simulink model "TireTestRig"  (R2020b)
settings: Solver=ode1  StartTime=0.0  StopTime=Tf  FixedStep=Ts  RelTol=1e-3  EnableMultiTasking=on
values from neighbouring files (symbols this model uses):
  Fz_forced = 1    [Main.m]
  p1 = 20    [Main.m]
  p2 = tire_data.UNLOADED_RADIUS    [Main.m]
  p3 = 9    [Main.m]
  p4 = 0.11    [Main.m]
  p5 = 6    [Main.m]
  p6 = tire_data.WIDTH/2    [Main.m]
  p7 = 1    [Main.m]
  p8 = 0    [Main.m]
  road_file = '../files_rdf/sample.rdf'    [Main.m]
  test_name = 'sine_thetaX'    [Main.m]
  tire_data = TIR_read('205_60_R15__left_debug.tir')    [Main.m]
  Ts = 1e-3    (= 0.001)    [Main.m]
undefined symbols (not defined in the file or in its folder): DiscIntNeverNeededParam, en_pressure, en_theta_x, en_theta_y, en_theta_z, en_x, en_y, en_z, inputs
libraries: RF_transformations x9, simulink x7, pid_lib x1, tire x1
settings Model: PacingRate=0.028000  Creator=matteolarcher  LastModifiedBy=matteolarcher
settings SolverCC: ConcurrentTasks=on
settings DataIOCC: SaveFormat=Array  ReturnWorkspaceOutputs=off

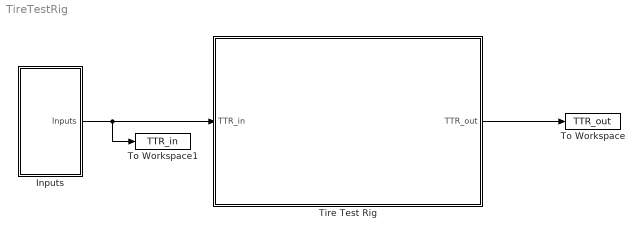
== system TireTestRig ==
  Inputs : Subsystem
  Tire Test Rig : Subsystem
  To Workspace : ToWorkspace  VariableName=TTR_out  SaveFormat=Timeseries  SampleTime=-1
  To Workspace1 : ToWorkspace  VariableName=TTR_in  SaveFormat=Timeseries  SampleTime=-1
  wires:
  Inputs/1(Inputs) -> To Workspace1/1, Tire Test Rig/1(TTR_in)
  Tire Test Rig/1(TTR_out) -> To Workspace/1

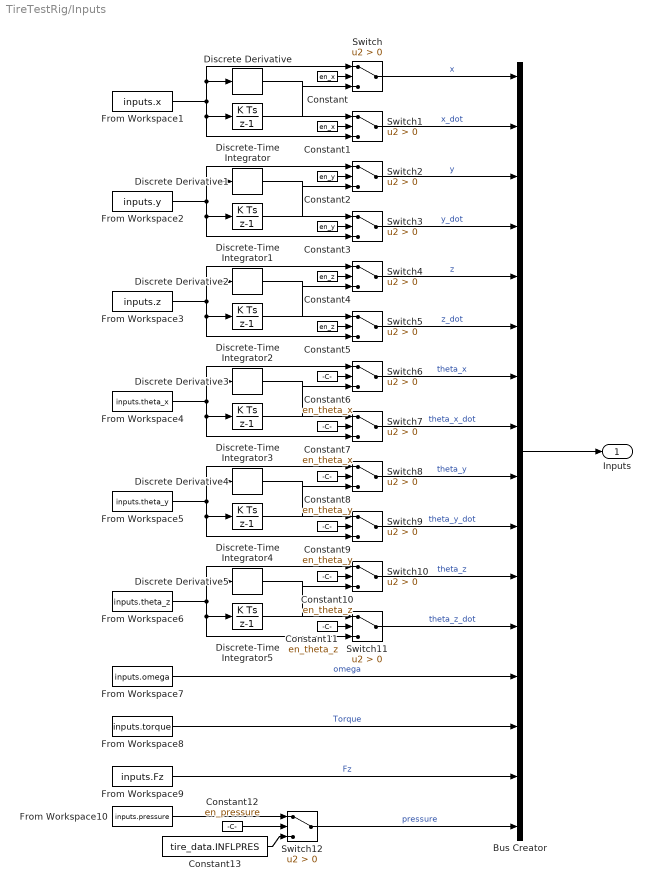
== system TireTestRig/Inputs ==
  Bus Creator : BusCreator  Inputs=16
  Constant : Constant  Value=en_x
  Constant1 : Constant  Value=en_x
  Constant10 : Constant  Value=en_theta_z
  Constant11 : Constant  Value=en_theta_z
  Constant12 : Constant  Value=en_pressure
  Constant13 : Constant  Value=tire_data.INFLPRES
  Constant2 : Constant  Value=en_y
  Constant3 : Constant  Value=en_y
  Constant4 : Constant  Value=en_z
  Constant5 : Constant  Value=en_z
  Constant6 : Constant  Value=en_theta_x
  Constant7 : Constant  Value=en_theta_x
  Constant8 : Constant  Value=en_theta_y
  Constant9 : Constant  Value=en_theta_y
  Discrete Derivative{,1..5} (6 alike) : simulink/Discrete/Discrete Derivative  gainval=1.0  ICPrevScaledInput=0.0  OutMin=[]  OutMax=[]  OutDataType=fixdt(1, 16)  OutScaling=2^-10  DoSatur=off
  Discrete-Time Integrator : DiscreteIntegrator  InitialCondition=inputs.x0  SampleTime=-1  ICPrevOutput=DiscIntNeverNeededParam  ICPrevScaledInput=DiscIntNeverNeededParam
  Discrete-Time Integrator1 : DiscreteIntegrator  InitialCondition=inputs.y0  SampleTime=-1  ICPrevOutput=DiscIntNeverNeededParam  ICPrevScaledInput=DiscIntNeverNeededParam
  Discrete-Time Integrator2 : DiscreteIntegrator  InitialCondition=inputs.z0  SampleTime=-1  ICPrevOutput=DiscIntNeverNeededParam  ICPrevScaledInput=DiscIntNeverNeededParam
  Discrete-Time Integrator3 : DiscreteIntegrator  InitialCondition=inputs.theta_x0  SampleTime=-1  ICPrevOutput=DiscIntNeverNeededParam  ICPrevScaledInput=DiscIntNeverNeededParam
  Discrete-Time Integrator4 : DiscreteIntegrator  InitialCondition=inputs.theta_y0  SampleTime=-1  ICPrevOutput=DiscIntNeverNeededParam  ICPrevScaledInput=DiscIntNeverNeededParam
  Discrete-Time Integrator5 : DiscreteIntegrator  InitialCondition=inputs.theta_z0  SampleTime=-1  ICPrevOutput=DiscIntNeverNeededParam  ICPrevScaledInput=DiscIntNeverNeededParam
  From Workspace1 : FromWorkspace  VariableName=inputs.x
  From Workspace10 : FromWorkspace  VariableName=inputs.pressure
  From Workspace2 : FromWorkspace  VariableName=inputs.y
  From Workspace3 : FromWorkspace  VariableName=inputs.z
  From Workspace4 : FromWorkspace  VariableName=inputs.theta_x
  From Workspace5 : FromWorkspace  VariableName=inputs.theta_y
  From Workspace6 : FromWorkspace  VariableName=inputs.theta_z
  From Workspace7 : FromWorkspace  VariableName=inputs.omega
  From Workspace8 : FromWorkspace  VariableName=inputs.torque
  From Workspace9 : FromWorkspace  VariableName=inputs.Fz
  Switch{,1..12} (13 alike) : Switch  Criteria=u2 > Threshold
  Inputs : Outport
  wires:
  Bus Creator/1 -> Inputs/1
  Switch/1 -> Bus Creator/1  "x"
  Discrete Derivative/1 -> Switch1/1
  Switch1/1 -> Bus Creator/2  "x_dot"
  From Workspace1/1 -> Switch/1, Discrete Derivative/1, Switch1/3, Discrete-Time Integrator/1
  Discrete-Time Integrator/1 -> Switch/3
  Constant/1 -> Switch/2
  Constant1/1 -> Switch1/2
  Constant3/1 -> Switch3/2
  Constant2/1 -> Switch2/2
  Discrete-Time Integrator1/1 -> Switch2/3
  From Workspace2/1 -> Discrete-Time Integrator1/1, Switch3/3, Discrete Derivative1/1, Switch2/1
  Switch3/1 -> Bus Creator/4  "y_dot"
  Discrete Derivative1/1 -> Switch3/1
  Switch2/1 -> Bus Creator/3  "y"
  Switch4/1 -> Bus Creator/5  "z"
  Discrete Derivative2/1 -> Switch5/1
  Switch5/1 -> Bus Creator/6  "z_dot"
  From Workspace3/1 -> Switch4/1, Discrete Derivative2/1, Switch5/3, Discrete-Time Integrator2/1
  Discrete-Time Integrator2/1 -> Switch4/3
  Constant4/1 -> Switch4/2
  Constant5/1 -> Switch5/2
  Constant11/1 -> Switch11/2
  Constant10/1 -> Switch10/2
  Discrete-Time Integrator5/1 -> Switch10/3
  From Workspace6/1 -> Discrete-Time Integrator5/1, Switch11/3, Discrete Derivative5/1, Switch10/1
  Switch11/1 -> Bus Creator/12  "theta_z_dot"
  Discrete Derivative5/1 -> Switch11/1
  Switch10/1 -> Bus Creator/11  "theta_z"
  Switch8/1 -> Bus Creator/9  "theta_y"
  Discrete Derivative4/1 -> Switch9/1
  Switch9/1 -> Bus Creator/10  "theta_y_dot"
  From Workspace5/1 -> Switch8/1, Discrete Derivative4/1, Switch9/3, Discrete-Time Integrator4/1
  Discrete-Time Integrator4/1 -> Switch8/3
  Constant8/1 -> Switch8/2
  Constant9/1 -> Switch9/2
  Constant7/1 -> Switch7/2
  Constant6/1 -> Switch6/2
  Discrete-Time Integrator3/1 -> Switch6/3
  From Workspace4/1 -> Discrete-Time Integrator3/1, Switch7/3, Discrete Derivative3/1, Switch6/1
  Switch7/1 -> Bus Creator/8  "theta_x_dot"
  Discrete Derivative3/1 -> Switch7/1
  Switch6/1 -> Bus Creator/7  "theta_x"
  From Workspace7/1 -> Bus Creator/13  "omega"
  From Workspace8/1 -> Bus Creator/14  "Torque"
  From Workspace9/1 -> Bus Creator/15  "Fz"
  From Workspace10/1 -> Switch12/1
  Constant12/1 -> Switch12/2
  Constant13/1 -> Switch12/3
  Switch12/1 -> Bus Creator/16  "pressure"

== system TireTestRig/Tire Test Rig ==
  note: in sin ThetaY anomalia pc e normale
      |
      | libreria macroblocchi
      |
      | controllo per 0 long slip
  TTR_in : Inport
  TTR_outputs : BusCreator  Inputs=3
  TireTestRig : Subsystem  TreatAsAtomicUnit=on
  TTR_out : Outport
  wires:
  TTR_outputs/1 -> TTR_out/1
  TTR_in/1 -> TireTestRig/1(inputs)
  TireTestRig/1(Tire Bus) -> TTR_outputs/1  "Tire Bus"
  TireTestRig/2(ENVE Bus) -> TTR_outputs/2  "ENVE Bus"
  TireTestRig/3(Actuator Bus) -> TTR_outputs/3  "Actuator Bus"

== system TireTestRig/Tire Test Rig/TireTestRig ==
  inputs : Inport
  ENVE : Subsystem
  Graphics : Subsystem
  Rig Actuator : Subsystem
  Tire : Subsystem
  Tire Bus : Outport
  ENVE Bus : Outport  Port=2
  Actuator Bus : Outport  Port=3
  wires:
  inputs/1 -> Tire/3(Inputs), Rig Actuator/2(inputs)
  Tire/1(Tire Bus) -> Graphics/1(Tire Bus), Tire Bus/1, Rig Actuator/1(tire Bus)
  Rig Actuator/1(Actuator Bus) -> Actuator Bus/1, Graphics/3(Actuator Bus), Tire/2(Actuator Bus), ENVE/1(Actuator Bus)
  ENVE/1(ENVE Bus) -> ENVE Bus/1, Graphics/2(ENVE Bus), Tire/1(ENVE Bus)

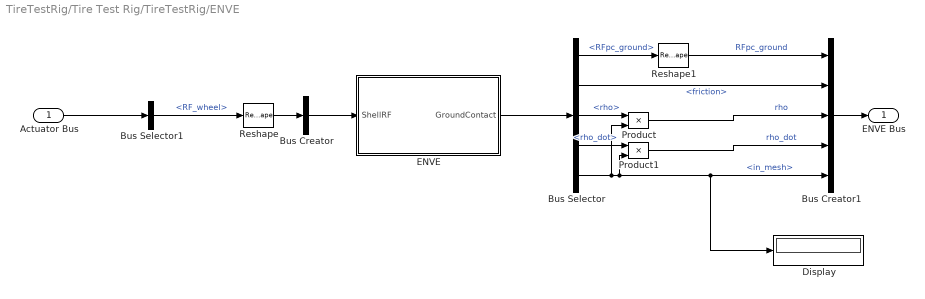
== system TireTestRig/Tire Test Rig/TireTestRig/ENVE ==
  Actuator Bus : Inport
  Bus Creator : BusCreator  Inputs=1  OutDataTypeStr=Bus: shellRF
      settings: InheritFromInputs=off
  Bus Creator1 : BusCreator  Inputs=5
  Bus Selector : BusSelector  OutputSignals=RFpc_ground,friction,rho,rho_dot,in_mesh
  Bus Selector1 : BusSelector  OutputSignals=RF_wheel
  Display : Display
  ENVE : Subsystem  mask{SParameter1=p1, SParameter2=p2, SParameter3=p3, SParameter4=p4, SParameter5=p5, SParameter6=p6, SParameter7=p7, SParameter8=p8}
      mask prompts: SParameter1 "Ribs number"; SParameter2 "Shell radius on x axis (m)"; SParameter3 "Shell curve degree for x axis"; SParameter4 "Shell radius on y axis (m)"; SParameter5 "Shell curve degree for y axis"; SParameter6 "Shell half width on y axis (m)"; SParameter7 "enveloping method"; SParameter8 "flat_enable"
      mask TypeOptions SParameter1: sfun_ENVE_VIRTUALTESTBENCH/SParameter1
      mask TypeOptions SParameter2: sfun_ENVE_VIRTUALTESTBENCH/SParameter2
      mask TypeOptions SParameter3: sfun_ENVE_VIRTUALTESTBENCH/SParameter3
      mask TypeOptions SParameter4: sfun_ENVE_VIRTUALTESTBENCH/SParameter4
      mask TypeOptions SParameter5: sfun_ENVE_VIRTUALTESTBENCH/SParameter5
      mask TypeOptions SParameter6: sfun_ENVE_VIRTUALTESTBENCH/SParameter6
      mask TypeOptions SParameter7: sfun_ENVE_VIRTUALTESTBENCH/SParameter7
      mask TypeOptions SParameter8: sfun_ENVE_VIRTUALTESTBENCH/SParameter8
  Product : Product
  Product1 : Product
  Reshape : Reshape
  Reshape1 : Reshape  OutputDimensionality=Customize  OutputDimensions=[4,4]
  ENVE Bus : Outport
  wires:
  Product1/1 -> Bus Creator1/4  "rho_dot"
  Bus Selector/5 -> Product/2, Display/1, Bus Creator1/5, Product1/2  "<in_mesh>"
  Reshape1/1 -> Bus Creator1/1  "RFpc_ground"
  Bus Creator/1 -> ENVE/1(ShellRF)
  Product/1 -> Bus Creator1/3  "rho"
  ENVE/1(GroundContact) -> Bus Selector/1
  Bus Selector/2 -> Bus Creator1/2  "<friction>"
  Bus Selector/1 -> Reshape1/1  "<RFpc_ground>"
  Actuator Bus/1 -> Bus Selector1/1
  Reshape/1 -> Bus Creator/1
  Bus Selector/3 -> Product/1  "<rho>"
  Bus Selector/4 -> Product1/1  "<rho_dot>"
  Bus Selector1/1 -> Reshape/1  "<RF_wheel>"
  Bus Creator1/1 -> ENVE Bus/1

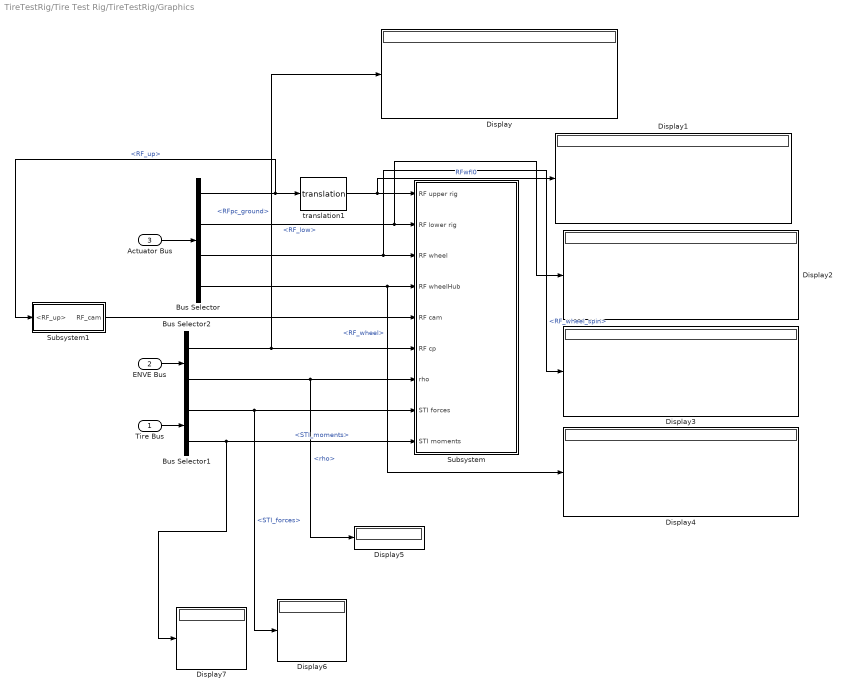
== system TireTestRig/Tire Test Rig/TireTestRig/Graphics ==
  Tire Bus : Inport
  ENVE Bus : Inport  Port=2
  Actuator Bus : Inport  Port=3
  Bus Selector : BusSelector  OutputSignals=RF_up,RF_low,RF_wheel_spin,RF_wheel
  Bus Selector1 : BusSelector  OutputSignals=STI_forces,STI_moments
  Bus Selector2 : BusSelector  OutputSignals=RFpc_ground,rho
  Display{,1..7} (8 alike) : Display
  Subsystem : Subsystem  mask{sample_time=Ts*100, tire_data=tire_data, road_file=road_file, rig_up_stl='rig_up.stl', rig_up_stl_scale=1e-3, rig_low_stl='rig_low.stl', rig_low_stl_scale=1e-3, wheel_stl={'SHELL',p1,p2,p3,p4,p5,p6}, wheel_stl_scale=1, en_trace_wheel=off, en_trace_cp=off, en_RF_wheel=on, en_RF_cp=on, en_RF_wheelHub=on, en_normal=on, en_forces=on, en_moments=on, save_gif=on, gif_folder=['./outputs/', test_name, '/GIF']}
      mask prompts: sample_time "sample time"; road_file "road file"; rig_up_stl "rig upper stl"; rig_up_stl_scale "rig upper stl scaling factor"; rig_low_stl "rig lower stl"; rig_low_stl_scale "rig lower stl scaling factor"; wheel_stl "wheel stl"; wheel_stl_scale "wheel stl scaling factor"; en_trace_wheel "enable wheel trace"; en_trace_cp "enable contact point trace"; en_RF_wheel "enable RF wheel"; en_RF_cp "enable RF contact point"; en_RF_wheelHub "enable RF wheel hub"; en_normal "enable normal vector"; en_forces "enable STI forces"; en_moments "enable STI moments"; save_gif "Save GIF"; gif_folder "GIF folder"
      mask init:
      | % create stl from shell geometry
      | if iscell(wheel_stl) && strcmp(wheel_stl{1}, 'SHELL')
      |     S = enve_shell(wheel_stl{2},wheel_stl{3},wheel_stl{4},wheel_stl{5},wheel_stl{6},wheel_stl{7});
      |     mesh = S.meshShell;
      |     surf2stl('./tmp/SHELL.stl',mesh.X,mesh.Y,mesh.Z,'ascii');
      |     wheel_stl = 'SHELL.stl';
      |     en_realdim_scaling = 0;
      | else
      |     en_realdim_scaling = 1;
      | end
      mask TypeOptions sample_time:
      | Level-2 MATLAB
      | S-Function1/sample_time
      mask TypeOptions tire_data:
      | Level-2 MATLAB
      | S-Function1/tire_data
      mask TypeOptions road_file:
      | Level-2 MATLAB
      | S-Function1/road_file
      mask TypeOptions rig_up_stl:
      | Level-2 MATLAB
      | S-Function1/rig_up_stl
      mask TypeOptions rig_up_stl_scale:
      | Level-2 MATLAB
      | S-Function1/rig_up_stl_scale
      mask TypeOptions rig_low_stl:
      | Level-2 MATLAB
      | S-Function1/rig_low_stl
      mask TypeOptions rig_low_stl_scale:
      | Level-2 MATLAB
      | S-Function1/rig_low_stl_scale
      mask TypeOptions wheel_stl:
      | Level-2 MATLAB
      | S-Function1/wheel_stl
      mask TypeOptions wheel_stl_scale:
      | Level-2 MATLAB
      | S-Function1/wheel_stl_scale
      mask TypeOptions en_trace_wheel:
      | Level-2 MATLAB
      | S-Function1/en_trace_wheel
      mask TypeOptions en_trace_cp:
      | Level-2 MATLAB
      | S-Function1/en_trace_cp
      mask TypeOptions en_RF_wheel:
      | Level-2 MATLAB
      | S-Function1/en_RF_wheel
      mask TypeOptions en_RF_cp:
      | Level-2 MATLAB
      | S-Function1/en_RF_cp
      mask TypeOptions en_RF_wheelHub:
      | Level-2 MATLAB
      | S-Function1/en_RF_wheelHub
      mask TypeOptions en_normal:
      | Level-2 MATLAB
      | S-Function1/en_normal
      mask TypeOptions en_forces:
      | Level-2 MATLAB
      | S-Function1/en_forces
      mask TypeOptions en_moments:
      | Level-2 MATLAB
      | S-Function1/en_moments
      mask TypeOptions save_gif:
      | Level-2 MATLAB
      | S-Function1/save_gif
      mask TypeOptions gif_folder:
      | Level-2 MATLAB
      | S-Function1/gif_folder
      mask DialogControl Container3 Prompt: GIF
  Subsystem1 : Subsystem  mask{xt=1, yt=-0, zt=0.2}
  translation1 : RF_transformations/translation  xt=0  yt=0.3+0.075  zt=0.3
  wires:
  Bus Selector/2 -> Display2/1, Subsystem/2(RF lower rig)  "<RF_low>"
  translation1/1 -> Display1/1, Subsystem/1(RF upper rig)  "RFwfl0"
  Bus Selector/3 -> Display3/1, Subsystem/3(RF wheel)  "<RF_wheel_spin>"
  Actuator Bus/1 -> Bus Selector/1
  Bus Selector/1 -> Subsystem1/1(<RF_up>), translation1/1  "<RF_up>"
  Tire Bus/1 -> Bus Selector1/1
  ENVE Bus/1 -> Bus Selector2/1
  Bus Selector2/1 -> Display/1, Subsystem/6(RF cp)  "<RFpc_ground>"
  Bus Selector2/2 -> Display5/1, Subsystem/7(rho)  "<rho>"
  Bus Selector1/1 -> Display6/1, Subsystem/8(STI forces)  "<STI_forces>"
  Bus Selector1/2 -> Display7/1, Subsystem/9(STI moments)  "<STI_moments>"
  Bus Selector/4 -> Display4/1, Subsystem/4(RF wheelHub)  "<RF_wheel>"
  Subsystem1/1(RF_cam) -> Subsystem/5(RF cam)

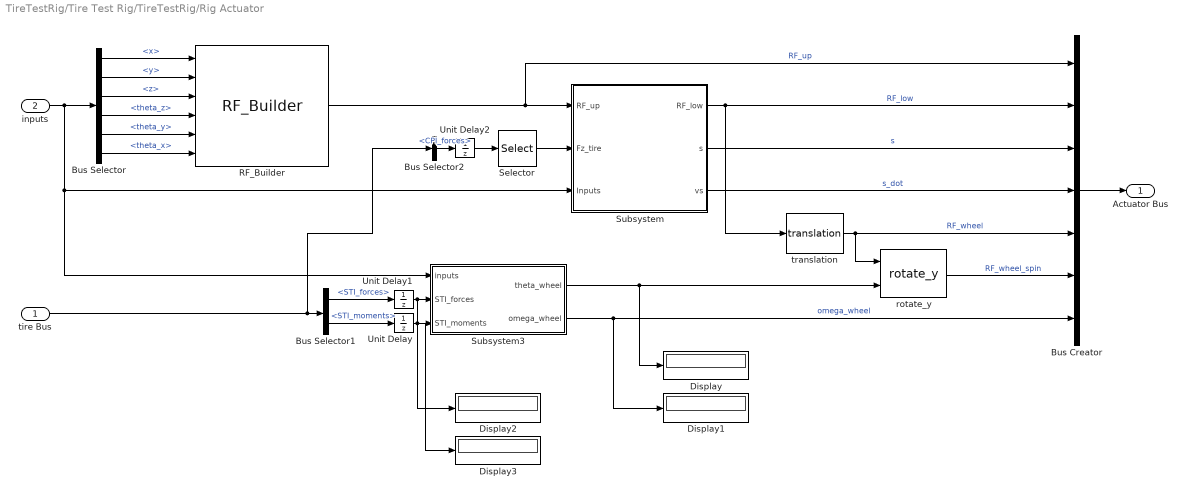
== system TireTestRig/Tire Test Rig/TireTestRig/Rig Actuator ==
  tire Bus : Inport
  inputs : Inport  Port=2
  Bus Creator : BusCreator  Inputs=7
  Bus Selector : BusSelector  OutputSignals=x,y,z,theta_z,theta_y,theta_x
  Bus Selector1 : BusSelector  OutputSignals=STI_forces,STI_moments
  Bus Selector2 : BusSelector  OutputSignals=CPI_forces
  Display{,1..3} (4 alike) : Display
  RF_Builder : RF_transformations/RF_Builder  order_selector=['Z','Y','X']
  Selector : Selector  InputPortWidth=3  IndexOptions=Index vector (dialog)  Indices=[3]  OutputSizes=1
  Subsystem : Subsystem  Variant=on  VariantControl=Choice
  Subsystem3 : Subsystem
  Unit Delay : UnitDelay  SampleTime=-1  HasFrameUpgradeWarning=on
  Unit Delay1 : UnitDelay  SampleTime=-1  HasFrameUpgradeWarning=on
  Unit Delay2 : UnitDelay  SampleTime=-1  HasFrameUpgradeWarning=on
  rotate_y : RF_transformations/rotate_y  SystemSampleTime=-1  VariantActivationTime=update diagram  Latency=0  AutoFrameSizeCalculation=off
  translation : RF_transformations/translation  xt=0  yt=0  zt=0
  Actuator Bus : Outport
  wires:
  Subsystem/2(s) -> Bus Creator/3  "s"
  Subsystem/3(vs) -> Bus Creator/4  "s_dot"
  Selector/1 -> Subsystem/2(Fz_tire)
  Subsystem/1(RF_low) -> translation/1, Bus Creator/2  "RF_low"
  Bus Selector2/1 -> Unit Delay2/1  "<CPI_forces>"
  RF_Builder/1 -> Subsystem/1(RF_up), Bus Creator/1  "RF_up"
  Bus Selector/5 -> RF_Builder/5  "<theta_y>"
  Bus Selector/4 -> RF_Builder/4  "<theta_z>"
  Bus Selector/6 -> RF_Builder/6  "<theta_x>"
  Bus Selector/3 -> RF_Builder/3  "<z>"
  Bus Selector/2 -> RF_Builder/2  "<y>"
  Bus Selector/1 -> RF_Builder/1  "<x>"
  inputs/1 -> Bus Selector/1, Subsystem3/1(inputs), Subsystem/3(Inputs)
  rotate_y/1 -> Bus Creator/6  "RF_wheel_spin"
  translation/1 -> rotate_y/1, Bus Creator/5  "RF_wheel"
  Subsystem3/1(theta_wheel) -> Display/1, rotate_y/2
  Subsystem3/2(omega_wheel) -> Display1/1, Bus Creator/7  "omega_wheel"
  Bus Selector1/2 -> Unit Delay/1  "<STI_moments>"
  Bus Selector1/1 -> Unit Delay1/1  "<STI_forces>"
  tire Bus/1 -> Bus Selector2/1, Bus Selector1/1
  Bus Creator/1 -> Actuator Bus/1
  Unit Delay/1 -> Display3/1, Subsystem3/3(STI_moments)
  Unit Delay1/1 -> Display2/1, Subsystem3/2(STI_forces)
  Unit Delay2/1 -> Selector/1

== system TireTestRig/Tire Test Rig/TireTestRig/Tire ==
  ENVE Bus : Inport
  Actuator Bus : Inport  Port=2
  Inputs : Inport  Port=3
  Bus Creator : BusCreator  Inputs=7
  Display : Display
  Display1 : Display
  Display2 : Display
  My_Tire_programmable : tire/My_Tire_programmable  Ts_tire=-1  tmp_tire_data=tire_data  enabled_rewind_tire=off  PauseResume=0  USE_MODE=tire_use_mode  pressure_from=tire pressure from input port  tire_p=1  Fz_flag=Fz_forced
  Subsystem1 : Subsystem
  Tire Bus : Outport
  wires:
  My_Tire_programmable/1 -> Bus Creator/1  "CPI_forces"
  My_Tire_programmable/2 -> Bus Creator/2  "CPI_moments"
  My_Tire_programmable/3 -> Bus Creator/3  "slips"
  My_Tire_programmable/4 -> Bus Creator/4  "STI_forces"
  My_Tire_programmable/5 -> Bus Creator/5  "STI_moments"
  Bus Creator/1 -> Tire Bus/1
  Inputs/1 -> Subsystem1/1(Inputs)
  ENVE Bus/1 -> Subsystem1/2(ENVE Bus)
  Actuator Bus/1 -> Subsystem1/3(Actuator Bus)
  Subsystem1/1(RFpc_groung) -> My_Tire_programmable/1
  Subsystem1/2(RF_wheel) -> Display2/1, My_Tire_programmable/2
  Subsystem1/3(vel) -> Bus Creator/6, My_Tire_programmable/3  "wheelHub_vel"
  Subsystem1/4(Omega) -> Bus Creator/7, My_Tire_programmable/4  "wheelHub_angVel"
  Subsystem1/5(omega_wheel) -> My_Tire_programmable/5
  Subsystem1/6(friction) -> My_Tire_programmable/6
  Subsystem1/7(rho/Fz) -> Display1/1, My_Tire_programmable/7
  Subsystem1/8(rho_dot) -> Display/1, My_Tire_programmable/8
  Subsystem1/9(pressure) -> My_Tire_programmable/9

== system TireTestRig/Tire Test Rig/TireTestRig/ENVE/ENVE ==
  ShellRF : Inport
  sfun_ENVE_VIRTUALTESTBENCH : S-Function  FunctionName=sfun_ENVE_VIRTUALTESTBENCH  Parameters=SParameter1, SParameter2, SParameter3, SParameter4, SParameter5, SParameter6, SParameter7, SParameter8  SFunctionDeploymentMode=off  EnableBusSupport=off  mask(Legacy Function){SFunctionSpec=void sfun_out(shellRF       u1[1], groundContact y1[1], double        p7[1], double        p8[1]), SParameter1=SParameter1, SParameter2=SParameter2, SParameter3=SParameter3, SParameter4=SParameter4, SParameter5=SParameter5, SParameter6=SParameter6, SParameter7=SParameter7, SParameter8=SParameter8, ShowSpec=off}
      mask prompts: SParameter1 "P1:"; SParameter2 "P2:"; SParameter3 "P3:"; SParameter4 "P4:"; SParameter5 "P5:"; SParameter6 "P6:"; SParameter7 "P7:"; SParameter8 "P8:"; ShowSpec "Display function specification"
      mask help:
      | This block allows you to call the legacy functions specified by the following Legacy Code Tool definition:
      | def.SFunctionName = 'sfun_ENVE_VIRTUALTESTBENCH';
      | def.OutputFcnSpec = 'void sfun_out(shellRFu1[1], groundContact y1[1], doublep7[1], doublep8[1]) ';
      | def.StartFcnSpec = 'void sfun_init(double p1[1], double p2[1], double p3[1], double p4[1], double p5[1], double p6[1]) ';
      | def.TerminateFcnSpec = 'void sfun_end()';
      | def.HeaderFiles = {'sfun_types.h', 'sfun_interface.h', 'sfun_shellVehicle.hh'};
      | def.SourceFiles = {'sfun_interface.cc', 'sfun_shellVehicle.cc'};
      | def.HostLibFiles = {'./../../lib/dll/libenve_osx.dylib'};
      | def.IncPaths = {'./include_sfun', './../src'};
      | def.SrcPaths = {'./src_sfun', './../src'};
      | def.LibPaths = {'./../../lib/dll'};
      mask Help: <p>This block was generated automatically by the Legacy Code Tool. For detailed help on this tool, call<a href="matlab:legacy_code('help')"> legacy_code('help')</a>.</p>
      mask Callback ShowSpec:
      | if strcmp(get_param(gcbh, 'ShowSpec'), 'on')
      |   set_param(gcbh, 'MaskDisplay', sprintf('fprintf(''%s'');', get_param(gcbh, 'SFunctionSpec')));
      | else
      |   set_param(gcbh, 'MaskDisplay', sprintf('fprintf(''%s'');', get_param(gcbh, 'FunctionName')));
      | end
      mask Display: fprintf('sfun_ENVE_VIRTUALTESTBENCH');
  GroundContact : Outport
  wires:
  ShellRF/1 -> sfun_ENVE_VIRTUALTESTBENCH/1
  sfun_ENVE_VIRTUALTESTBENCH/1 -> GroundContact/1

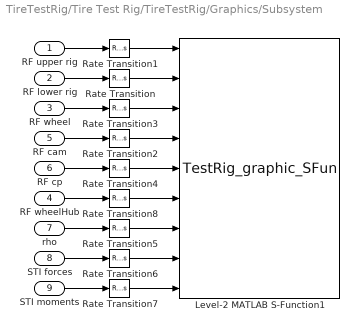
== system TireTestRig/Tire Test Rig/TireTestRig/Graphics/Subsystem ==
  RF upper rig : Inport
  RF lower rig : Inport  Port=2
  RF wheel : Inport  Port=3
  RF wheelHub : Inport  Port=4
  RF cam : Inport  Port=5
  RF cp : Inport  Port=6
  rho : Inport  Port=7
  STI forces : Inport  Port=8
  STI moments : Inport  Port=9
  Level-2 MATLAB S-Function1 : M-S-Function  FunctionName=TestRig_graphic_SFun  Parameters=sample_time tire_data road_file rig_up_stl rig_up_stl_scale rig_low_stl rig_low_stl_scale wheel_stl wheel_stl_scale en_realdim_scaling en_trace_wheel en_trace_cp en_RF_wheel en_RF_cp en_RF_wheelHub en_normal en_forces en_moments save_gif gif_folder  mask{sample_time=sample_time, tire_data=tire_data, road_file=road_file, rig_up_stl=rig_up_stl, rig_up_stl_scale=rig_up_stl_scale, rig_low_stl=rig_low_stl, rig_low_stl_scale=rig_low_stl_scale, wheel_stl=wheel_stl, wheel_stl_scale=wheel_stl_scale, en_trace_wheel=off, en_trace_cp=off, en_RF_wheel=on, en_RF_cp=on, en_RF_wheelHub=on, en_normal=on, en_forces=on, en_moments=on, save_gif=on, gif_folder=gif_folder}
      mask prompts: sample_time "sample time"; road_file "road file"; rig_up_stl "rig upper stl"; rig_up_stl_scale "rig upper stl scaling factor"; rig_low_stl "rig lower stl"; rig_low_stl_scale "rig lower stl scaling factor"; wheel_stl "wheel stl"; wheel_stl_scale "wheel stl scaling factor"; en_trace_wheel "enable wheel trace"; en_trace_cp "enable contact point trace"; en_RF_wheel "enable RF wheel"; en_RF_cp "enable RF contact point"; en_RF_wheelHub "enable RF wheel hub"; en_normal "enable normal vector"; en_forces "enable STI forces"; en_moments "enable STI moments"; save_gif "Save GIF"; gif_folder "GIF folder"
      mask Callback save_gif:
      | A = get_param(gcb,'save_gif');
      | m = Simulink.Mask.get(gcb);
      | 
      | p1 = m.getParameter('gif_folder');
      | 
      | if strcmp(A, 'on')
      |     p1.Enabled = 'on';
      | else
      |     p1.Enabled = 'off';
      | end
      mask DialogControl Container3 Prompt: GIF
  Rate Transition{,1..4,8} (6 alike) : RateTransition  Deterministic=off  InitialCondition=eye(4)  OutPortSampleTimeOpt=Inherit
  Rate Transition5 : RateTransition  Deterministic=off  OutPortSampleTimeOpt=Inherit
  Rate Transition6 : RateTransition  Deterministic=off  InitialCondition=[0 0 0]  OutPortSampleTimeOpt=Inherit
  Rate Transition7 : RateTransition  Deterministic=off  InitialCondition="[0 0  0]"  OutPortSampleTimeOpt=Inherit
  wires:
  RF cam/1 -> Rate Transition2/1
  RF lower rig/1 -> Rate Transition/1
  RF upper rig/1 -> Rate Transition1/1
  Rate Transition2/1 -> Level-2 MATLAB S-Function1/4
  Rate Transition/1 -> Level-2 MATLAB S-Function1/2
  Rate Transition1/1 -> Level-2 MATLAB S-Function1/1
  RF wheel/1 -> Rate Transition3/1
  Rate Transition3/1 -> Level-2 MATLAB S-Function1/3
  RF cp/1 -> Rate Transition4/1
  rho/1 -> Rate Transition5/1
  STI forces/1 -> Rate Transition6/1
  STI moments/1 -> Rate Transition7/1
  Rate Transition4/1 -> Level-2 MATLAB S-Function1/5
  Rate Transition5/1 -> Level-2 MATLAB S-Function1/7
  Rate Transition6/1 -> Level-2 MATLAB S-Function1/8
  Rate Transition7/1 -> Level-2 MATLAB S-Function1/9
  RF wheelHub/1 -> Rate Transition8/1
  Rate Transition8/1 -> Level-2 MATLAB S-Function1/6

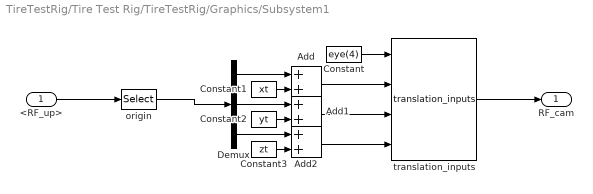
== system TireTestRig/Tire Test Rig/TireTestRig/Graphics/Subsystem1 ==
  <RF_up> : Inport
  Add : Sum
  Add1 : Sum
  Add2 : Sum
  Constant : Constant  Value=eye(4)
  Constant1 : Constant  Value=xt
  Constant2 : Constant  Value=yt
  Constant3 : Constant  Value=zt
  Demux : Demux  Outputs=3
  origin : Selector  NumberOfDimensions=2  InputPortWidth=3  IndexOptions=Index vector (dialog),Index vector (dialog)  Indices=[1 2 3],[4]  OutputSizes=1,1
  translation_inputs : RF_transformations/translation_inputs  SystemSampleTime=-1  VariantActivationTime=update diagram  Latency=0  AutoFrameSizeCalculation=off
  RF_cam : Outport
  wires:
  <RF_up>/1 -> origin/1
  Constant2/1 -> Add1/2
  Constant3/1 -> Add2/2
  Demux/3 -> Add2/1
  Demux/2 -> Add1/1
  Demux/1 -> Add/1
  Constant/1 -> translation_inputs/1
  Constant1/1 -> Add/2
  translation_inputs/1 -> RF_cam/1
  origin/1 -> Demux/1
  Add/1 -> translation_inputs/2
  Add1/1 -> translation_inputs/3
  Add2/1 -> translation_inputs/4

== system TireTestRig/Tire Test Rig/TireTestRig/Rig Actuator/Subsystem ==
  RF_up : Inport
  Fz_tire : Inport  Port=2
  Inputs : Inport  Port=3
  Controlled_Fz_loop : Subsystem  VariantControl=actuation_type == 4
  Controlled_Fz_pid : Subsystem  VariantControl=actuation_type == 3
  Fixed : Subsystem  VariantControl=actuation_type == 1
  Spring : Subsystem  VariantControl=actuation_type == 2
  RF_low : Outport
  s : Outport  Port=2
  vs : Outport  Port=3

== system TireTestRig/Tire Test Rig/TireTestRig/Rig Actuator/Subsystem3 ==
  inputs : Inport
  STI_forces : Inport  Port=2
  STI_moments : Inport  Port=3
  Bus Selector : BusSelector  OutputSignals=omega,Torque
  Selector : Selector  InputPortWidth=3  IndexOptions=Index vector (dialog)  Indices=[1]  OutputSizes=1
  Selector1 : Selector  InputPortWidth=3  IndexOptions=Index vector (dialog)  Indices=[2]  OutputSizes=1
  Subsystem : Subsystem  Variant=on  VariantControl=Choice
  theta_wheel : Outport
  omega_wheel : Outport  Port=2
  wires:
  Subsystem/2(theta) -> theta_wheel/1
  Subsystem/1(omega_out) -> omega_wheel/1
  Selector1/1 -> Subsystem/4(my_tire)
  STI_moments/1 -> Selector1/1
  Selector/1 -> Subsystem/3(fx_tire)
  STI_forces/1 -> Selector/1
  Bus Selector/2 -> Subsystem/2(torque)  "<Torque>"
  Bus Selector/1 -> Subsystem/1(omega_in)  "<omega>"
  inputs/1 -> Bus Selector/1

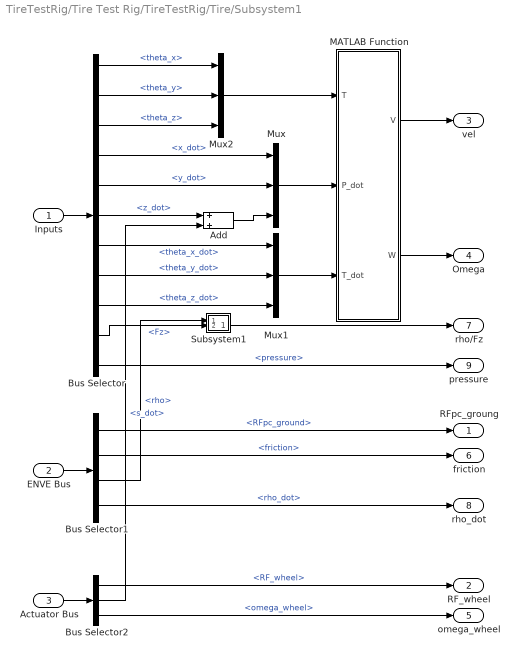
== system TireTestRig/Tire Test Rig/TireTestRig/Tire/Subsystem1 ==
  Inputs : Inport
  ENVE Bus : Inport  Port=2
  Actuator Bus : Inport  Port=3
  Add : Sum
  Bus Selector : BusSelector  OutputSignals=theta_x,theta_y,theta_z,x_dot,y_dot,z_dot,theta_x_dot,theta_y_dot,theta_z_dot,Fz,pressure
  Bus Selector1 : BusSelector  OutputSignals=RFpc_ground,friction,rho,rho_dot
  Bus Selector2 : BusSelector  OutputSignals=RF_wheel,s_dot,omega_wheel
  MATLAB Function : MATLAB Function  TreatAsAtomicUnit=on
  Mux : Mux  Inputs=3
  Mux1 : Mux  Inputs=3
  Mux2 : Mux  Inputs=3
  Subsystem1 : Subsystem
  RFpc_groung : Outport
  RF_wheel : Outport  Port=2
  vel : Outport  Port=3
  Omega : Outport  Port=4
  omega_wheel : Outport  Port=5
  friction : Outport  Port=6
  rho/Fz : Outport  Port=7
  rho_dot : Outport  Port=8
  pressure : Outport  Port=9
  wires:
  Bus Selector/6 -> Add/1  "<z_dot>"
  Mux1/1 -> MATLAB Function/3(T_dot)
  Inputs/1 -> Bus Selector/1
  Add/1 -> Mux/3
  Bus Selector/8 -> Mux1/2  "<theta_y_dot>"
  Mux/1 -> MATLAB Function/2(P_dot)
  Bus Selector/5 -> Mux/2  "<y_dot>"
  Bus Selector/7 -> Mux1/1  "<theta_x_dot>"
  Bus Selector/9 -> Mux1/3  "<theta_z_dot>"
  Bus Selector/4 -> Mux/1  "<x_dot>"
  Bus Selector2/3 -> omega_wheel/1  "<omega_wheel>"
  Actuator Bus/1 -> Bus Selector2/1
  Bus Selector1/3 -> Subsystem1/1(rho)  "<rho>"
  Bus Selector2/1 -> RF_wheel/1  "<RF_wheel>"
  ENVE Bus/1 -> Bus Selector1/1
  Bus Selector1/1 -> RFpc_groung/1  "<RFpc_ground>"
  Bus Selector2/2 -> Add/2  "<s_dot>"
  Bus Selector1/2 -> friction/1  "<friction>"
  Bus Selector1/4 -> rho_dot/1  "<rho_dot>"
  Bus Selector/10 -> Subsystem1/2(Fz)  "<Fz>"
  Subsystem1/1(Out1) -> rho/Fz/1
  Bus Selector/11 -> pressure/1  "<pressure>"
  Bus Selector/1 -> Mux2/1  "<theta_x>"
  Bus Selector/2 -> Mux2/2  "<theta_y>"
  Bus Selector/3 -> Mux2/3  "<theta_z>"
  MATLAB Function/2(W) -> Omega/1
  MATLAB Function/1(V) -> vel/1
  Mux2/1 -> MATLAB Function/1(T)

== system TireTestRig/Tire Test Rig/TireTestRig/Rig Actuator/Subsystem/Controlled_Fz_loop ==
  RF_up : Inport
  Fz_tire : Inport  Port=2
  Inputs : Inport  Port=3
  Constant : Constant
  Constant1 : Constant  Value=0
  MATLAB Function : MATLAB Function  TreatAsAtomicUnit=on
  Terminator : Terminator
  While Iterator Subsystem : Subsystem  TreatAsAtomicUnit=on
  RF_low : Outport
  s : Outport  Port=2
  vs : Outport  Port=3
  wires:
  Constant/1 -> While Iterator Subsystem/3(IC)
  RF_up/1 -> While Iterator Subsystem/1(RF_in)
  Inputs/1 -> While Iterator Subsystem/2(Inputs)
  While Iterator Subsystem/2(s) -> s/1
  While Iterator Subsystem/1(RF_out) -> RF_low/1
  Constant1/1 -> vs/1
  Fz_tire/1 -> Terminator/1
  While Iterator Subsystem/3(Fz_warning) -> MATLAB Function/1(Fz_warning)
  While Iterator Subsystem/4(Fz_error) -> MATLAB Function/2(Fz_error)

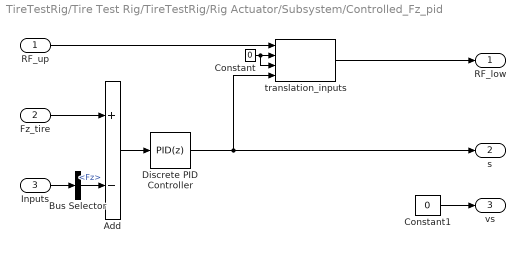
== system TireTestRig/Tire Test Rig/TireTestRig/Rig Actuator/Subsystem/Controlled_Fz_pid ==
  RF_up : Inport
  Fz_tire : Inport  Port=2
  Inputs : Inport  Port=3
  Add : Sum  Inputs=+-
  Bus Selector : BusSelector  OutputSignals=Fz
  Constant : Constant  Value=0
  Constant1 : Constant  Value=0
  Discrete PID Controller : pid_lib/PID Controller  Controller=PID  Form=Parallel  TimeDomain=Discrete-time  UseExternalTs=off  SampleTime=-1  IntegratorMethod=Forward Euler  FilterMethod=Forward Euler  ControllerParametersSource=internal  P=1/tire_data.VERTICAL_STIFFNESS  I=1e-4  D=0  UseFilter=on  N=100  TunerSelectOption=Transfer Function Based (PID Tuner App)  InitialConditionSource=internal  InitialConditionForIntegrator=0  InitialConditionForFilter=0  DifferentiatorICPrevScaledInput=0  ExternalReset=none  TrackingMode=off  Kt=1  LimitOutput=off  SatLimitsSource=internal  UpperSaturationLimit=inf  LowerSaturationLimit=-inf  LinearizeAsGain=off  AntiWindupMode=none  Kb=1  POutMin=[]  POutMax=[]  IOutMin=[]  IOutMax=[]  DOutMin=[]  DOutMax=[]  NOutMin=[]  NOutMax=[]  SumOutMin=[]  SumOutMax=[]  SaturationOutMin=[]  SaturationOutMax=[]  PParamMin=[]  PParamMax=[]  IParamMin=[]  IParamMax=[]  DParamMin=[]  DParamMax=[]  NParamMin=[]  NParamMax=[]  KbParamMin=[]  KbParamMax=[]  KtParamMin=[]  KtParamMax=[]  KbOutMin=[]  KbOutMax=[]  KtOutMin=[]  KtOutMax=[]  IntegratorOutMin=[]  IntegratorOutMax=[]  FilterOutMin=[]  FilterOutMax=[]  SumI1OutMin=[]  SumI1OutMax=[]  SumI2OutMin=[]  SumI2OutMax=[]  SumI3OutMin=[]  SumI3OutMax=[]  SumI4OutMin=[]  SumI4OutMax=[]  SumDOutMin=[]  SumDOutMax=[]  DifferentiatorOutMin=[]  DifferentiatorOutMax=[]  FilterDiffOutCoefMin=[]  FilterDiffOutCoefMax=[]  ReciprocalOutMin=[]  ReciprocalOutMax=[]  SumDenOutMin=[]  SumDenOutMax=[]  SumNumOutMin=[]  SumNumOutMax=[]  DivideOutMin=[]  DivideOutMax=[]  UdiffTsProdOutMin=[]  UdiffTsProdOutMax=[]  NTsProdOutMin=[]  NTsProdOutMax=[]  UintegralTsProdOutMin=[]  UintegralTsProdOutMax=[]  UngainTsProdOutMin=[]  UngainTsProdOutMax=[]  IntegratorContinuousStateAttributes=''  IntegratorStateMustResolveToSignalObject=off  IntegratorRTWStateStorageClass=Auto  FilterContinuousStateAttributes=''  FilterStateMustResolveToSignalObject=off  FilterRTWStateStorageClass=Auto  ParallelPVariant=InternalParameters  IdealPVariant=Disabled  IVariant=InternalParameters  DVariant=InternalParameters  IntegratorVariant=Discrete  SatVariant=Disabled  AWVariant=Passthrough  PCopyVariant=Disabled  TRVariant=Disabled  FdbkBlocksVariant=Forward  IdealPFdbkVariant=Disabled  SatFdbkVariant=Disabled  DerivativeFilterVariant=ForwardEulerFilter  NVariant=InternalParameters  NCopyVariant=Disabled  FilterICVariant=InternalICsFilter  IntegratorICVariant=InternalICs  ExternalResetVariant=Disabled  TRSumVariant=Passthrough  SumFdbkVariant=Disabled  SumVariant=Sum_PID  TsampFilterVariant=InternalTs  TsampNgainVariant=Passthrough  TsampIntegralVariant=Passthrough  ExternalSaturationOutDataTypeStr=Inherit: Same as second input
  translation_inputs : RF_transformations/translation_inputs  SystemSampleTime=-1  VariantActivationTime=update diagram  Latency=0  AutoFrameSizeCalculation=off
  RF_low : Outport
  s : Outport  Port=2
  vs : Outport  Port=3
  wires:
  Bus Selector/1 -> Add/2  "<Fz>"
  Fz_tire/1 -> Add/1
  Discrete PID Controller/1 -> translation_inputs/4, s/1
  Add/1 -> Discrete PID Controller/1
  Constant1/1 -> vs/1
  Inputs/1 -> Bus Selector/1
  Constant/1 -> translation_inputs/2, translation_inputs/3
  translation_inputs/1 -> RF_low/1
  RF_up/1 -> translation_inputs/1

== system TireTestRig/Tire Test Rig/TireTestRig/Rig Actuator/Subsystem/Fixed ==
  RF_up : Inport
  Fz_tire : Inport  Port=2
  Inputs : Inport  Port=3
  Constant : Constant  Value=0
  Terminator : Terminator
  Terminator1 : Terminator
  RF_low : Outport
  s : Outport  Port=2
  vs : Outport  Port=3
  wires:
  Constant/1 -> s/1, vs/1
  RF_up/1 -> RF_low/1
  Inputs/1 -> Terminator1/1
  Fz_tire/1 -> Terminator/1

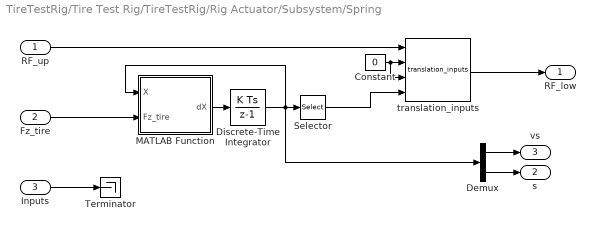
== system TireTestRig/Tire Test Rig/TireTestRig/Rig Actuator/Subsystem/Spring ==
  RF_up : Inport
  Fz_tire : Inport  Port=2
  Inputs : Inport  Port=3
  Constant : Constant  Value=0
  Demux : Demux  Outputs=2
  Discrete-Time Integrator : DiscreteIntegrator  SampleTime=-1  ICPrevOutput=DiscIntNeverNeededParam  ICPrevScaledInput=DiscIntNeverNeededParam
  MATLAB Function : MATLAB Function  TreatAsAtomicUnit=on  mask{k_spring=2000, damping=1000, preload=0.5, mass=20}
      mask prompts: k_spring "spring stiffness"; damping "damping coefficient"; mass "moving mass"
  Selector : Selector  InputPortWidth=2  IndexOptions=Index vector (dialog)  Indices=[2]  OutputSizes=1
  Terminator : Terminator
  translation_inputs : RF_transformations/translation_inputs  SystemSampleTime=-1  VariantActivationTime=update diagram  Latency=0  AutoFrameSizeCalculation=off
  RF_low : Outport
  s : Outport  Port=2
  vs : Outport  Port=3
  wires:
  Demux/1 -> vs/1
  Demux/2 -> s/1
  Constant/1 -> translation_inputs/2, translation_inputs/3
  Selector/1 -> translation_inputs/4
  RF_up/1 -> translation_inputs/1
  Inputs/1 -> Terminator/1
  translation_inputs/1 -> RF_low/1
  Fz_tire/1 -> MATLAB Function/2(Fz_tire)
  Discrete-Time Integrator/1 -> MATLAB Function/1(X), Selector/1, Demux/1
  MATLAB Function/1(dX) -> Discrete-Time Integrator/1

== system TireTestRig/Tire Test Rig/TireTestRig/Rig Actuator/Subsystem3/Subsystem ==
  omega_in : Inport
  torque : Inport  Port=2
  fx_tire : Inport  Port=3
  my_tire : Inport  Port=4
  Torque : Subsystem  VariantControl=en_torque == 1
  omega : Subsystem  VariantControl=en_torque == 0
  omega_out : Outport
  theta : Outport  Port=2

== system TireTestRig/Tire Test Rig/TireTestRig/Tire/Subsystem1/Subsystem1 ==
  rho : Inport
  Fz : Inport  Port=2
  Constant : Constant  Value=Fz_forced
  Switch : Switch  Criteria=u2 > Threshold
  Out1 : Outport
  wires:
  Fz/1 -> Switch/1
  Switch/1 -> Out1/1
  rho/1 -> Switch/3
  Constant/1 -> Switch/2

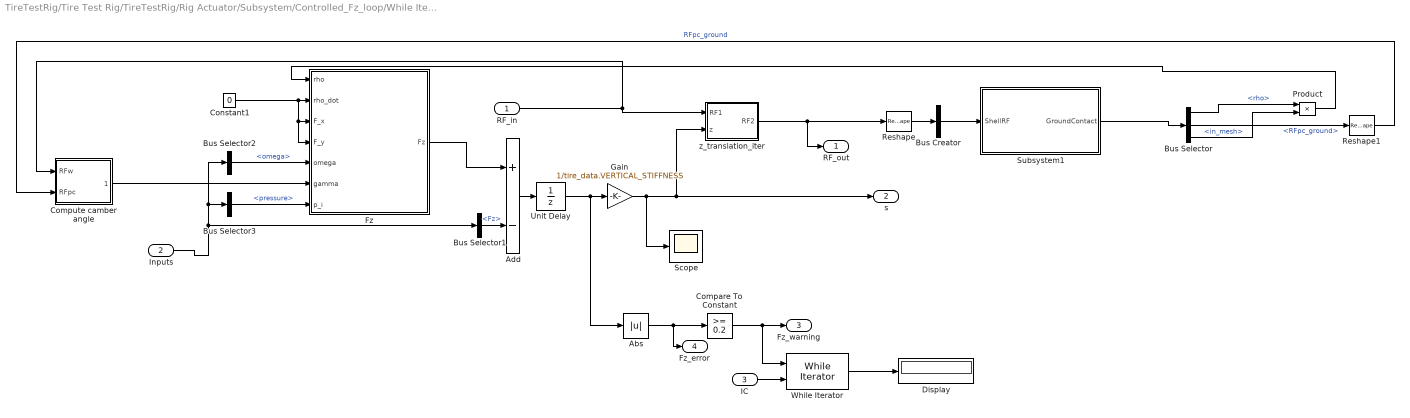
== system TireTestRig/Tire Test Rig/TireTestRig/Rig Actuator/Subsystem/Controlled_Fz_loop/While Iterator Subsystem ==
  RF_in : Inport
  Inputs : Inport  Port=2
  IC : Inport  Port=3
  Abs : Abs
  Add : Sum  Inputs=+-
  Bus Creator : BusCreator  Inputs=1  OutDataTypeStr=Bus: shellRF
      settings: InheritFromInputs=off
  Bus Selector : BusSelector  OutputSignals=rho,RFpc_ground,in_mesh
  Bus Selector1 : BusSelector  OutputSignals=Fz
  Bus Selector2 : BusSelector  OutputSignals=omega
  Bus Selector3 : BusSelector  OutputSignals=pressure
  Compare To Constant : simulink/Logic and Bit Operations/Compare To Constant  relop=>=  const=0.2  OutDataTypeStr=boolean
  Compute camber angle : Subsystem
  Constant1 : Constant  Value=0
  Display : Display
  Fz : MATLAB Function  TreatAsAtomicUnit=on  mask{tmp_tire_data=tire_data}
      mask prompts: tmp_tire_data "tire data"
      mask init:
      | % Keep only the numeric fields (avoir Simulink errors) and save it into parameterStruct
      | fn = fieldnames(tmp_tire_data);
      | for k = 1:numel(fn)
      |     v = tmp_tire_data.(fn{k});
      |     if(isnumeric(v))
      |         tire_data.(fn{k}) = v;
      |     end
      | end
  Gain : Gain  Gain=1/tire_data.VERTICAL_STIFFNESS
  Product : Product
  Reshape : Reshape
  Reshape1 : Reshape  OutputDimensionality=Customize  OutputDimensions=[4,4]
  Scope : Scope
  Subsystem1 : Subsystem  mask{SParameter1=p1, SParameter2=p2, SParameter3=p3, SParameter4=p4, SParameter5=p5, SParameter6=p6, SParameter7=p7, SParameter8=p8}
      mask prompts: SParameter1 "Ribs number"; SParameter2 "Shell radius on x axis (m)"; SParameter3 "Shell curve degree for x axis"; SParameter4 "Shell radius on y axis (m)"; SParameter5 "Shell curve degree for y axis"; SParameter6 "Shell half width on y axis (m)"; SParameter7 "enveloping method"; SParameter8 "flat_enable"
      mask TypeOptions SParameter1: sfun_ENVE_VIRTUALTESTBENCH/SParameter1
      mask TypeOptions SParameter2: sfun_ENVE_VIRTUALTESTBENCH/SParameter2
      mask TypeOptions SParameter3: sfun_ENVE_VIRTUALTESTBENCH/SParameter3
      mask TypeOptions SParameter4: sfun_ENVE_VIRTUALTESTBENCH/SParameter4
      mask TypeOptions SParameter5: sfun_ENVE_VIRTUALTESTBENCH/SParameter5
      mask TypeOptions SParameter6: sfun_ENVE_VIRTUALTESTBENCH/SParameter6
      mask TypeOptions SParameter7: sfun_ENVE_VIRTUALTESTBENCH/SParameter7
      mask TypeOptions SParameter8: sfun_ENVE_VIRTUALTESTBENCH/SParameter8
  Unit Delay : UnitDelay  SampleTime=-1  HasFrameUpgradeWarning=on
  While Iterator : WhileIterator  MaxIters=500  ShowIterationPort=on
  z_translation_iter : MATLAB Function  TreatAsAtomicUnit=on
  RF_out : Outport
  s : Outport  Port=2
  Fz_warning : Outport  Port=3
  Fz_error : Outport  Port=4
  wires:
  Bus Selector/1 -> Product/1  "<rho>"
  Bus Selector/3 -> Product/2  "<in_mesh>"
  Abs/1 -> Fz_error/1, Compare To Constant/1
  Reshape1/1 -> Compute camber angle/2(RFpc)  "RFpc_ground"
  Product/1 -> Fz/1(rho)
  Bus Selector/2 -> Reshape1/1  "<RFpc_ground>"
  Unit Delay/1 -> Gain/1, Abs/1
  Subsystem1/1(GroundContact) -> Bus Selector/1
  While Iterator/1 -> Display/1
  z_translation_iter/1(RF2) -> Reshape/1, RF_out/1
  Bus Selector3/1 -> Fz/7(p_i)  "<pressure>"
  Compute camber angle/1(gamma) -> Fz/6(gamma)
  Bus Selector2/1 -> Fz/5(omega)  "<omega>"
  Constant1/1 -> Fz/2(rho_dot), Fz/3(F_x), Fz/4(F_y)
  RF_in/1 -> Compute camber angle/1(RFw), z_translation_iter/1(RF1)
  Bus Selector1/1 -> Add/2  "<Fz>"
  Compare To Constant/1 -> Fz_warning/1, While Iterator/1
  Fz/1(Fz) -> Add/1
  Reshape/1 -> Bus Creator/1
  Bus Creator/1 -> Subsystem1/1(ShellRF)
  Gain/1 -> Scope/1, s/1, z_translation_iter/2(z)
  Inputs/1 -> Bus Selector3/1, Bus Selector2/1, Bus Selector1/1
  Add/1 -> Unit Delay/1
  IC/1 -> While Iterator/2

== system TireTestRig/Tire Test Rig/TireTestRig/Rig Actuator/Subsystem3/Subsystem/Torque ==
  omega_in : Inport
  torque : Inport  Port=2
  fx_tire : Inport  Port=3
  my_tire : Inport  Port=4
  Demux : Demux  Outputs=2
  Discrete-Time Integrator : DiscreteIntegrator  InitialCondition=[inputs.omega0, 0]  SampleTime=-1  ICPrevOutput=DiscIntNeverNeededParam  ICPrevScaledInput=DiscIntNeverNeededParam
  MATLAB Function : MATLAB Function  TreatAsAtomicUnit=on  mask{inertia=1, radius=tire_data.UNLOADED_RADIUS}
      mask prompts: inertia "wheel inertia"; radius "tire radius"
  Terminator : Terminator
  omega_out : Outport
  theta : Outport  Port=2
  wires:
  omega_in/1 -> Terminator/1
  Demux/2 -> theta/1
  Demux/1 -> omega_out/1
  Discrete-Time Integrator/1 -> MATLAB Function/1(X), Demux/1
  my_tire/1 -> MATLAB Function/4(My)
  fx_tire/1 -> MATLAB Function/3(Fx)
  torque/1 -> MATLAB Function/2(T)
  MATLAB Function/1(dX) -> Discrete-Time Integrator/1

== system TireTestRig/Tire Test Rig/TireTestRig/Rig Actuator/Subsystem3/Subsystem/omega ==
  omega_in : Inport
  torque : Inport  Port=2
  fx_tire : Inport  Port=3
  my_tire : Inport  Port=4
  Discrete-Time Integrator : DiscreteIntegrator  SampleTime=-1  ICPrevOutput=DiscIntNeverNeededParam  ICPrevScaledInput=DiscIntNeverNeededParam
  Terminator : Terminator
  Terminator1 : Terminator
  Terminator2 : Terminator
  omega_out : Outport
  theta : Outport  Port=2
  wires:
  Discrete-Time Integrator/1 -> theta/1
  my_tire/1 -> Terminator2/1
  fx_tire/1 -> Terminator1/1
  torque/1 -> Terminator/1
  omega_in/1 -> omega_out/1, Discrete-Time Integrator/1

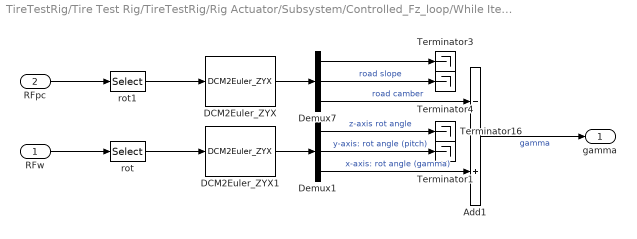
== system TireTestRig/Tire Test Rig/TireTestRig/Rig Actuator/Subsystem/Controlled_Fz_loop/While Iterator Subsystem/Compute camber angle ==
  RFw : Inport
  RFpc : Inport  Port=2
  Add1 : Sum  Inputs=-+
  DCM2Euler_ZYX : RF_transformations/DCM2Euler_ZYX  SystemSampleTime=-1  VariantActivationTime=update diagram  Latency=0  AutoFrameSizeCalculation=off
  DCM2Euler_ZYX1 : RF_transformations/DCM2Euler_ZYX  SystemSampleTime=-1  VariantActivationTime=update diagram  Latency=0  AutoFrameSizeCalculation=off
  Demux1 : Demux  Outputs=3
  Demux7 : Demux  Outputs=3
  Terminator{1,3..4,16} (4 alike) : Terminator
  rot : Selector  NumberOfDimensions=2  InputPortWidth=3  IndexOptions=Index vector (dialog),Index vector (dialog)  Indices=[1 2 3],[1 2 3]  OutputSizes=1,1
  rot1 : Selector  NumberOfDimensions=2  InputPortWidth=3  IndexOptions=Index vector (dialog),Index vector (dialog)  Indices=[1 2 3],[1 2 3]  OutputSizes=1,1
  gamma : Outport
  wires:
  RFpc/1 -> rot1/1
  Demux7/2 -> Terminator4/1  "road slope"
  Demux7/3 -> Add1/1  "road camber"
  rot1/1 -> DCM2Euler_ZYX/1
  RFw/1 -> rot/1
  DCM2Euler_ZYX/1 -> Demux7/1
  Add1/1 -> gamma/1  "gamma"
  rot/1 -> DCM2Euler_ZYX1/1
  Demux1/2 -> Terminator1/1  "y-axis: rot angle (pitch)"
  DCM2Euler_ZYX1/1 -> Demux1/1
  Demux1/1 -> Terminator16/1  "z-axis rot angle"
  Demux7/1 -> Terminator3/1
  Demux1/3 -> Add1/2  "x-axis: rot angle (gamma)"

== system TireTestRig/Tire Test Rig/TireTestRig/Rig Actuator/Subsystem/Controlled_Fz_loop/While Iterator Subsystem/Subsystem1 ==
  ShellRF : Inport
  sfun_ENVE_VIRTUALTESTBENCH : S-Function  FunctionName=sfun_ENVE_VIRTUALTESTBENCH  Parameters=SParameter1, SParameter2, SParameter3, SParameter4, SParameter5, SParameter6, SParameter7, SParameter8  SFunctionDeploymentMode=off  EnableBusSupport=off  mask(Legacy Function){SFunctionSpec=void sfun_out(shellRF       u1[1], groundContact y1[1], double        p7[1], double        p8[1]), SParameter1=SParameter1, SParameter2=SParameter2, SParameter3=SParameter3, SParameter4=SParameter4, SParameter5=SParameter5, SParameter6=SParameter6, SParameter7=SParameter7, SParameter8=SParameter8, ShowSpec=off}
      mask prompts: SParameter1 "P1:"; SParameter2 "P2:"; SParameter3 "P3:"; SParameter4 "P4:"; SParameter5 "P5:"; SParameter6 "P6:"; SParameter7 "P7:"; SParameter8 "P8:"; ShowSpec "Display function specification"
      mask help:
      | This block allows you to call the legacy functions specified by the following Legacy Code Tool definition:
      | def.SFunctionName = 'sfun_ENVE_VIRTUALTESTBENCH';
      | def.OutputFcnSpec = 'void sfun_out(shellRFu1[1], groundContact y1[1], doublep7[1], doublep8[1]) ';
      | def.StartFcnSpec = 'void sfun_init(double p1[1], double p2[1], double p3[1], double p4[1], double p5[1], double p6[1]) ';
      | def.TerminateFcnSpec = 'void sfun_end()';
      | def.HeaderFiles = {'sfun_types.h', 'sfun_interface.h', 'sfun_shellVehicle.hh'};
      | def.SourceFiles = {'sfun_interface.cc', 'sfun_shellVehicle.cc'};
      | def.HostLibFiles = {'./../../lib/dll/libenve_osx.dylib'};
      | def.IncPaths = {'./include_sfun', './../src'};
      | def.SrcPaths = {'./src_sfun', './../src'};
      | def.LibPaths = {'./../../lib/dll'};
      mask Help: <p>This block was generated automatically by the Legacy Code Tool. For detailed help on this tool, call<a href="matlab:legacy_code('help')"> legacy_code('help')</a>.</p>
      mask Callback ShowSpec:
      | if strcmp(get_param(gcbh, 'ShowSpec'), 'on')
      |   set_param(gcbh, 'MaskDisplay', sprintf('fprintf(''%s'');', get_param(gcbh, 'SFunctionSpec')));
      | else
      |   set_param(gcbh, 'MaskDisplay', sprintf('fprintf(''%s'');', get_param(gcbh, 'FunctionName')));
      | end
      mask Display: fprintf('sfun_ENVE_VIRTUALTESTBENCH');
  GroundContact : Outport
  wires:
  sfun_ENVE_VIRTUALTESTBENCH/1 -> GroundContact/1
  ShellRF/1 -> sfun_ENVE_VIRTUALTESTBENCH/1

== matlab function TireTestRig/Tire Test Rig/TireTestRig/Tire/Subsystem1/MATLAB Function ==
  data: T input; V output; P_dot input; T_dot input; W output
function [V,W] = fcn(T,P_dot, T_dot)

theta__x = T(1);
theta__y = T(2);
theta__z = T(3);

x__dot = P_dot(1);
y__dot = P_dot(2);
z__dot = P_dot(3);

theta__x__dot = T_dot(1);
theta__y__dot = T_dot(2);
theta__z__dot = T_dot(3);

vx = cos(theta__y) * x__dot * cos(theta__z) + cos(theta__y) * y__dot * sin(theta__z) - z__dot * sin(theta__y);
vy = (-sin(theta__z) * cos(theta__x) + cos(theta__z) * sin(theta__y) * sin(theta__x)) * x__dot + (cos(theta__z) * cos(theta__x) + sin(theta__z) * sin(theta__y) * sin(theta__x)) * y__dot + cos(theta__y) * z__dot * sin(theta__x);
vz = (sin(theta__z) * sin(theta__x) + cos(theta__z) * sin(theta__y) * cos(theta__x)) * x__dot + (-cos(theta__z) * sin(theta__x) + sin(theta__z) * sin(theta__y) * cos(theta__x)) * y__dot + cos(theta__y) * cos(theta__x) * z__dot;

wx = -theta__z__dot * sin(theta__y) + theta__x__dot;
wy = sin(theta__x) * cos(theta__y) * theta__z__dot + theta__y__dot * cos(theta__x);
wz = cos(theta__x) * cos(theta__y) * theta__z__dot - theta__y__dot * sin(theta__x);

V = [vx,vy,vz]';
W = [wx,wy,wz]';

== matlab function TireTestRig/Tire Test Rig/TireTestRig/Rig Actuator/Subsystem/Controlled_Fz_loop/MATLAB Function ==
  data: Fz_warning input; Fz_error input
function fcn(Fz_warning, Fz_error)

if Fz_warning
    error('Fz has not converged to the desired value. Fz error is: %d N', Fz_error);
end

== matlab function TireTestRig/Tire Test Rig/TireTestRig/Rig Actuator/Subsystem/Controlled_Fz_loop/While Iterator Subsystem/Fz ==
  data: rho input; rho_dot input; F_x input; F_y input; omega input; gamma input; p_i input; Fz output; tire_data parameter
function Fz = fcn(rho,rho_dot,F_x,F_y,omega,gamma,p_i,tire_data)

% initialize tire class !!! TEMPORARY WORKAROUND !!!
if tire_data.FITTYP == 62
    TIRE = pacejka_model_62_class(tire_data, 0);
    Fz = TIRE.compute_F_z(rho, rho_dot, omega, gamma, p_i, F_x, F_y);
elseif tire_data.FITTYP == 52
    TIRE = pacejka_model_52_class(tire_data, 0);
    Fz = TIRE.compute_F_z(rho, rho_dot, omega, gamma, p_i, F_x, F_y);
else
    Fz = NaN;
end

end

== matlab function TireTestRig/Tire Test Rig/TireTestRig/Rig Actuator/Subsystem/Controlled_Fz_loop/While Iterator Subsystem/z_translation_iter ==
  data: RF1 input size=[4,4]; RF2 output size=[4,4]; z input
function RF2 = translation(RF1, z)

persistent z_t

if isempty(z_t)
    z_t = z;
    
else
    z_t = z_t + z;
end

RF2 = RF1*(eye(4) + [zeros(4,3) [0,0,z_t,0]']);

end

== matlab function TireTestRig/Tire Test Rig/TireTestRig/Rig Actuator/Subsystem/Spring/MATLAB Function ==
  data: X input; Fz_tire input; dX output size=[2]; k_spring parameter; damping parameter; mass parameter; preload parameter
function dX = fcn(X, Fz_tire,k_spring, damping, mass, preload)



dx1 = (Fz_tire - k_spring * (X(2) + preload) - damping * X(1))/ mass;
dx2 = X(1);

dX = [dx1; dx2];

== matlab function TireTestRig/Tire Test Rig/TireTestRig/Rig Actuator/Subsystem3/Subsystem/Torque/MATLAB Function ==
  data: X input; dX output; T input; Fx input; My input; inertia parameter; radius parameter
function dX = fcn(X, T, Fx, My, inertia, radius)

dx1 = (T- Fx * radius + My) / inertia;

dx2 = X(1);

dX = [dx1, dx2];
